simulink model "scd3busMicrogridDroopControlFidelityLevels"  (R2025b)
settings: Solver=ode15s  StartTime=0.0  StopTime=48  RelTol=1e-3
PreLoadFcn:
  | scd3busMicrogridDroopControlDataFidelityLevels;
  | 
  | %% Controller variants
  | % Create variant controls for converter controller. Controller has two
  | % different levels of fidelity: Averaged, AveragedPulse, Pulse
  | Averaged = Simulink.VariantExpression;
  | Averaged.Condition = 'fidelity==scd3busMicrogridDroopControl_variants_enum.Low';
  | Pulse = Simulink.VariantExpression;
  | Pulse.Condition = 'fidelity==scd3busMicrogridDroopControl_variants_enum.High';
  | 
  | %% Plant variants
  | % Create variant controls for converter plant. Plant has three different
  | % levels of fidelity.
  | AveragedNonSwitch = Simulink.VariantExpression;
  | AveragedNonSwitch.Condition = 'fidelity==scd3busMicrogridDroopControl_variants_enum.Low';
  | PulseSwitch = Simulink.VariantExpression;
  | PulseSwitch.Condition = 'fidelity==scd3busMicrogridDroopControl_variants_enum.High';
  | 
  | %% Set up variables ready for simulation
  | fidelity = scd3busMicrogridDroopControl_variants_enum.High;
  | Ts = 5e-6;
  | Ts_V = 1e-6;
  | Tsc = 1e-4;
  | Tsc_V = 5e-4;
values from neighbouring files (symbols this model uses):
  consensus = 1    [scd3busMicrogridDroopControlDataFidelityLevels.m]
  fgrid = 60    [scd3busMicrogridDroopControlDataFidelityLevels.m]    (also in scd3busMicrogridDroopControlDataFidelityLevels3Inv.m)
  Kdroop_fp = 0.02/2    (= 0.01)    [scd3busMicrogridDroopControlDataFidelityLevels.m]
  Kdroop_vq = 0.02/2    (= 0.01)    [scd3busMicrogridDroopControlDataFidelityLevels.m]
  Ki_vd = 850    [scd3busMicrogridDroopControlDataFidelityLevels.m]    (also in scd3busMicrogridDroopControlDataFidelityLevels3Inv.m)
  Ki_vq = 850    [scd3busMicrogridDroopControlDataFidelityLevels.m]    (also in scd3busMicrogridDroopControlDataFidelityLevels3Inv.m)
  Kp_vd = 0.36    [scd3busMicrogridDroopControlDataFidelityLevels.m]    (also in scd3busMicrogridDroopControlDataFidelityLevels3Inv.m)
  Kp_vq = 0.36    [scd3busMicrogridDroopControlDataFidelityLevels.m]    (also in scd3busMicrogridDroopControlDataFidelityLevels3Inv.m)
  Ts_DC = 0.001    [scd3busMicrogridDroopControlDataFidelityLevels.m]    (also in scd3busMicrogridDroopControlDataFidelityLevels3Inv.m = 0.0001)
  Vdc1 = 1000    [scd3busMicrogridDroopControlDataFidelityLevels.m]    (also in scd3busMicrogridDroopControlDataFidelityLevels3Inv.m)
  Vdc2 = 1000    [scd3busMicrogridDroopControlDataFidelityLevels.m]    (also in scd3busMicrogridDroopControlDataFidelityLevels3Inv.m)
  Vrms = 380    [scd3busMicrogridDroopControlDataFidelityLevels.m]    (also in scd3busMicrogridDroopControlDataFidelityLevels3Inv.m)
libraries: nesl_utility x60, ee_lib x57, fl_lib x32, eeTransforms x8, eeSinusoidalMeasurement x8, slpidlib x8, eePwmGeneratorTwoLevel x4, eePowerMeasurement x4, simulink x4, SignalEditorBlockLib x1
(part 2 of 5)

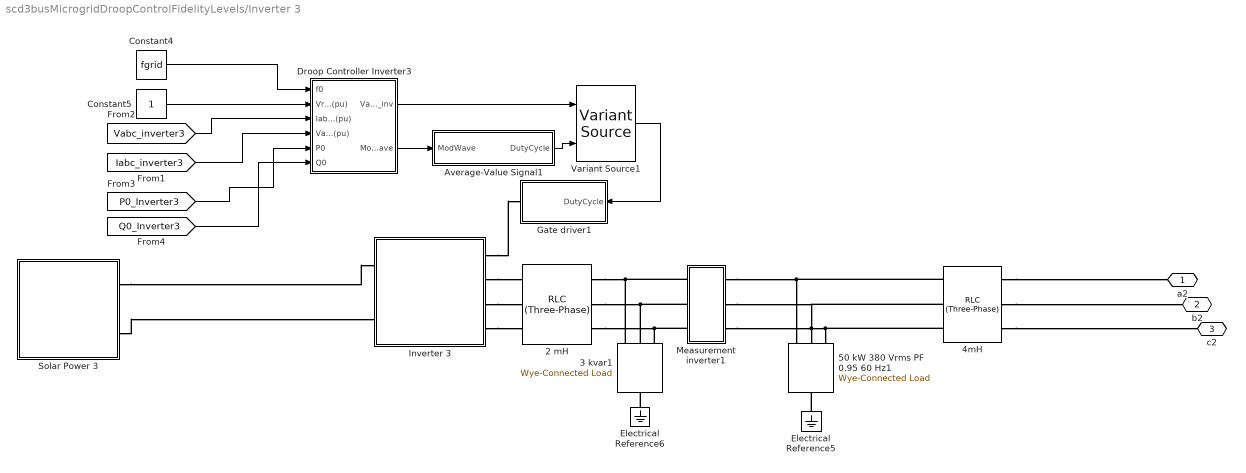
== system scd3busMicrogridDroopControlFidelityLevels/Inverter 3 ==
  2 mH : ee_lib/Passive/RLC Assemblies/RLC (Three-Phase)  port_option=ee.enum.threePhasePort.expanded  component_structure=ee.enum.rlc.structure.SeriesRL  R=0.02 Ohm  L=0.002 H  C=1 F  R_parasitic=1e-6 Ohm  G_parasitic=1e-6 1/Ohm  IL_specify=on  IL_priority=High  IL=[0, 0, 0] A  IL_nominal_specify=off  IL_nominal_value=1  IL_nominal_unit=A  VC_specify=on  VC_priority=High  VC=[0, 0, 0] V  VC_nominal_specify=off  VC_nominal_value=1  VC_nominal_unit=V
      settings: InternalSimscapePortConfiguration="{\"Bottom\":[],\"Left\":[{\"id\":\"a1\",\"label\":\"a1\",\"type\":\"foundation.electrical.electrical\"},{\"id\":\"b1\",\"label\":\"b1\",\"type\":\"foundation.electrical.electrical\"},{\"id\":\"c1\",\"label\":\"c1\",\"type\":\"foundation.electrical.electrical\"}],\"Right\":[{\"id\":\"a2\",\"label\":\"a2\",\"type\":\"foundation.electrical.electrical\"},{\"id\":\"b2\",\"label\":\"b2\",\"type\":\"foundation.electrical.electrical\"},{\"id\":\"c2\",\"label\":\"c2\",\"type\":\"foundation.electrical.electrical\"}],\"Top\":[]}"
  3 kvar1 : ee_lib/Passive/RLC Assemblies/Wye-Connected Load  port_option=ee.enum.threePhasePort.expanded  parameterization=ee.enum.rlc.parameterization.ratedpower  component_structure=ee.enum.rlc.structure.C  component_structure_PQ=ee.enum.rlc.structure.C  R=1 Ohm  L=0.001 H  C=1e-6 F  VRated=Vrms V  FRated=fgrid Hz  P=0 W  Qpos=0 A*V  Qneg=-3000 A*V  R_parasitic=1e-6 Ohm  G_parasitic=1e-6 1/Ohm  R_parasitic_PQ=1e-6 Ohm  G_parasitic_PQ=1e-6 1/Ohm  Vmag0=380 V  Vang0=0 deg  Freq0=60 Hz  IL_specify=on  IL_priority=High  IL=[ 0 0 0 ] A  IL_nominal_specify=off  IL_nominal_value=1  IL_nominal_unit=A  VC_specify=on  VC_priority=High  VC=[ 0 0 0 ] V  VC_nominal_specify=off  VC_nominal_value=1  VC_nominal_unit=V
      settings: InternalSimscapePortConfiguration="{\"Bottom\":[],\"Left\":[{\"id\":\"a\",\"label\":\"a\",\"type\":\"foundation.electrical.electrical\"},{\"id\":\"b\",\"label\":\"b\",\"type\":\"foundation.electrical.electrical\"},{\"id\":\"c\",\"label\":\"c\",\"type\":\"foundation.electrical.electrical\"}],\"Right\":[{\"id\":\"n\",\"label\":\"n\",\"type\":\"foundation.electrical.electrical\"}],\"Top\":[]}"
  "4mH " : ee_lib/Passive/RLC Assemblies/RLC (Three-Phase)  port_option=ee.enum.threePhasePort.expanded  component_structure=ee.enum.rlc.structure.SeriesRL  R=0.025 Ohm  L=0.004 H  C=1 F  R_parasitic=1e-6 Ohm  G_parasitic=1e-6 1/Ohm  IL_specify=on  IL_priority=High  IL=[0, 0, 0] A  IL_nominal_specify=off  IL_nominal_value=1  IL_nominal_unit=A  VC_specify=on  VC_priority=High  VC=[0, 0, 0] V  VC_nominal_specify=off  VC_nominal_value=1  VC_nominal_unit=V
      settings: InternalSimscapePortConfiguration="{\"Bottom\":[],\"Left\":[{\"id\":\"a1\",\"label\":\"a1\",\"type\":\"foundation.electrical.electrical\"},{\"id\":\"b1\",\"label\":\"b1\",\"type\":\"foundation.electrical.electrical\"},{\"id\":\"c1\",\"label\":\"c1\",\"type\":\"foundation.electrical.electrical\"}],\"Right\":[{\"id\":\"a2\",\"label\":\"a2\",\"type\":\"foundation.electrical.electrical\"},{\"id\":\"b2\",\"label\":\"b2\",\"type\":\"foundation.electrical.electrical\"},{\"id\":\"c2\",\"label\":\"c2\",\"type\":\"foundation.electrical.electrical\"}],\"Top\":[]}"
  50 kW 380 Vrms PF 0.95 60 Hz1 : ee_lib/Passive/RLC Assemblies/Wye-Connected Load  port_option=ee.enum.threePhasePort.expanded  parameterization=2  component_structure=1  component_structure_PQ=ee.enum.rlc.structure.ParallelRL  R=1 Ohm  L=0.001 H  C=1e-6 F  VRated=Vrms V  FRated=fgrid Hz  P=50000 W  Qpos=50000*sqrt(1-0.95^2)/0.95 V*A  Qneg=-3000 V*A  R_parasitic=1e-6 Ohm  G_parasitic=1e-6 1/Ohm  R_parasitic_PQ=1e-6 Ohm  G_parasitic_PQ=1e-6 1/Ohm  Vmag0=380 V  Vang0=0 deg  Freq0=60 Hz  IL_specify=on  IL_priority=High  IL=[ 0 0 0 ] A  IL_nominal_specify=off  IL_nominal_value=1  IL_nominal_unit=A  VC_specify=on  VC_priority=High  VC=[ 0 0 0 ] V  VC_nominal_specify=off  VC_nominal_value=1  VC_nominal_unit=V
      settings: InternalSimscapePortConfiguration="{\"Bottom\":[],\"Left\":[{\"id\":\"a\",\"label\":\"a\",\"type\":\"foundation.electrical.electrical\"},{\"id\":\"b\",\"label\":\"b\",\"type\":\"foundation.electrical.electrical\"},{\"id\":\"c\",\"label\":\"c\",\"type\":\"foundation.electrical.electrical\"}],\"Right\":[{\"id\":\"n\",\"label\":\"n\",\"type\":\"foundation.electrical.electrical\"}],\"Top\":[]}"
  Average-Value Signal1 : Subsystem
  Constant4 : Constant  Value=fgrid
  Constant5 : Constant
  Droop Controller Inverter3 : Subsystem
  Electrical Reference5 : fl_lib/Electrical/Electrical Elements/Electrical Reference
  Electrical Reference6 : fl_lib/Electrical/Electrical Elements/Electrical Reference
  Gate driver1 : Subsystem
  Inverter 3 : Subsystem  Variant=on  VariantControl=Choice
  Measurement inverter1 : Subsystem
  Solar Power 3 : Subsystem
  Variant Source1 : VariantSource  ShowConditionOnBlock=on  VariantControls={Pulse, Averaged}
  a2 : PMIOPort  Side=Right
  b2 : PMIOPort  Port=2  Side=Right
  c2 : PMIOPort  Port=3  Side=Right
  wires:
  Variant Source1/1 -> Gate driver1/1(DutyCycle)
  Droop Controller Inverter3/2(ModWave) -> Average-Value Signal1/1(ModWave)
  [P0_Inverter3] -> Droop Controller Inverter3/5(P0)
  [Vabc_inverter3] -> Droop Controller Inverter3/3(Iabc (pu))
  Constant4/1 -> Droop Controller Inverter3/1(f0)
  Constant5/1 -> Droop Controller Inverter3/2(Vref (pu))
  [Iabc_inverter3] -> Droop Controller Inverter3/4(Vabc (pu))
  Droop Controller Inverter3/1(Vabc_inv) -> Variant Source1/1
  [Q0_Inverter3] -> Droop Controller Inverter3/6(Q0)
  Average-Value Signal1/1(DutyCycle) -> Variant Source1/2
  connections:
  50 kW 380 Vrms PF 0.95 60 Hz1/LConn2 -- Measurement inverter1/RConn2 -- "4mH "/LConn2
  50 kW 380 Vrms PF 0.95 60 Hz1/LConn3 -- Measurement inverter1/RConn3 -- "4mH "/LConn3
  "4mH "/RConn1 -- a2/RConn1
  Inverter 3/LConn3 -- 2 mH/LConn2
  "4mH "/LConn1 -- Measurement inverter1/RConn1 -- 50 kW 380 Vrms PF 0.95 60 Hz1/LConn1
  Solar Power 3/RConn2 -- Inverter 3/RConn2
  "4mH "/RConn3 -- c2/RConn1
  Electrical Reference6/LConn1 -- 3 kvar1/RConn1
  Inverter 3/LConn4 -- 2 mH/LConn3
  "4mH "/RConn2 -- b2/RConn1
  Electrical Reference5/LConn1 -- 50 kW 380 Vrms PF 0.95 60 Hz1/RConn1
  2 mH/RConn2 -- Measurement inverter1/LConn2 -- 3 kvar1/LConn2
  2 mH/RConn3 -- Measurement inverter1/LConn3 -- 3 kvar1/LConn3
  Solar Power 3/RConn1 -- Inverter 3/RConn1
  2 mH/RConn1 -- Measurement inverter1/LConn1 -- 3 kvar1/LConn1
  Inverter 3/LConn2 -- 2 mH/LConn1
  Inverter 3/LConn1 -- Gate driver1/RConn1

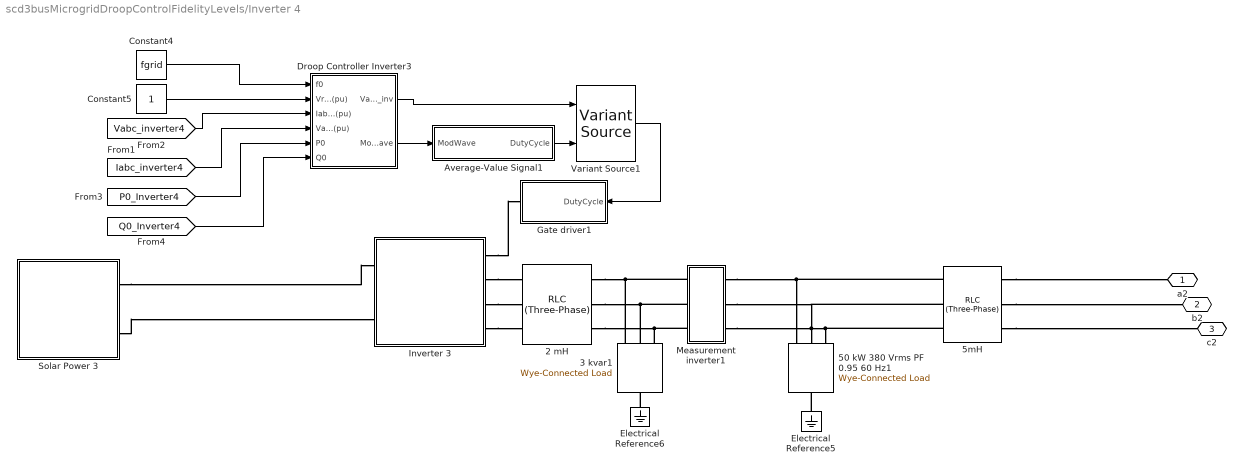
== system scd3busMicrogridDroopControlFidelityLevels/Inverter 4 ==
  2 mH : ee_lib/Passive/RLC Assemblies/RLC (Three-Phase)  port_option=ee.enum.threePhasePort.expanded  component_structure=ee.enum.rlc.structure.SeriesRL  R=0.02 Ohm  L=0.002 H  C=1 F  R_parasitic=1e-6 Ohm  G_parasitic=1e-6 1/Ohm  IL_specify=on  IL_priority=High  IL=[0, 0, 0] A  IL_nominal_specify=off  IL_nominal_value=1  IL_nominal_unit=A  VC_specify=on  VC_priority=High  VC=[0, 0, 0] V  VC_nominal_specify=off  VC_nominal_value=1  VC_nominal_unit=V
      settings: InternalSimscapePortConfiguration="{\"Bottom\":[],\"Left\":[{\"id\":\"a1\",\"label\":\"a1\",\"type\":\"foundation.electrical.electrical\"},{\"id\":\"b1\",\"label\":\"b1\",\"type\":\"foundation.electrical.electrical\"},{\"id\":\"c1\",\"label\":\"c1\",\"type\":\"foundation.electrical.electrical\"}],\"Right\":[{\"id\":\"a2\",\"label\":\"a2\",\"type\":\"foundation.electrical.electrical\"},{\"id\":\"b2\",\"label\":\"b2\",\"type\":\"foundation.electrical.electrical\"},{\"id\":\"c2\",\"label\":\"c2\",\"type\":\"foundation.electrical.electrical\"}],\"Top\":[]}"
  3 kvar1 : ee_lib/Passive/RLC Assemblies/Wye-Connected Load  port_option=ee.enum.threePhasePort.expanded  parameterization=ee.enum.rlc.parameterization.ratedpower  component_structure=ee.enum.rlc.structure.C  component_structure_PQ=ee.enum.rlc.structure.C  R=1 Ohm  L=0.001 H  C=1e-6 F  VRated=Vrms V  FRated=fgrid Hz  P=0 W  Qpos=0 A*V  Qneg=-3000 A*V  R_parasitic=1e-6 Ohm  G_parasitic=1e-6 1/Ohm  R_parasitic_PQ=1e-6 Ohm  G_parasitic_PQ=1e-6 1/Ohm  Vmag0=380 V  Vang0=0 deg  Freq0=60 Hz  IL_specify=on  IL_priority=High  IL=[ 0 0 0 ] A  IL_nominal_specify=off  IL_nominal_value=1  IL_nominal_unit=A  VC_specify=on  VC_priority=High  VC=[ 0 0 0 ] V  VC_nominal_specify=off  VC_nominal_value=1  VC_nominal_unit=V
      settings: InternalSimscapePortConfiguration="{\"Bottom\":[],\"Left\":[{\"id\":\"a\",\"label\":\"a\",\"type\":\"foundation.electrical.electrical\"},{\"id\":\"b\",\"label\":\"b\",\"type\":\"foundation.electrical.electrical\"},{\"id\":\"c\",\"label\":\"c\",\"type\":\"foundation.electrical.electrical\"}],\"Right\":[{\"id\":\"n\",\"label\":\"n\",\"type\":\"foundation.electrical.electrical\"}],\"Top\":[]}"
  50 kW 380 Vrms PF 0.95 60 Hz1 : ee_lib/Passive/RLC Assemblies/Wye-Connected Load  port_option=ee.enum.threePhasePort.expanded  parameterization=2  component_structure=1  component_structure_PQ=ee.enum.rlc.structure.ParallelRL  R=1 Ohm  L=0.001 H  C=1e-6 F  VRated=Vrms V  FRated=fgrid Hz  P=50000 W  Qpos=50000*sqrt(1-0.95^2)/0.95 V*A  Qneg=-3000 V*A  R_parasitic=1e-6 Ohm  G_parasitic=1e-6 1/Ohm  R_parasitic_PQ=1e-6 Ohm  G_parasitic_PQ=1e-6 1/Ohm  Vmag0=380 V  Vang0=0 deg  Freq0=60 Hz  IL_specify=on  IL_priority=High  IL=[ 0 0 0 ] A  IL_nominal_specify=off  IL_nominal_value=1  IL_nominal_unit=A  VC_specify=on  VC_priority=High  VC=[ 0 0 0 ] V  VC_nominal_specify=off  VC_nominal_value=1  VC_nominal_unit=V
      settings: InternalSimscapePortConfiguration="{\"Bottom\":[],\"Left\":[{\"id\":\"a\",\"label\":\"a\",\"type\":\"foundation.electrical.electrical\"},{\"id\":\"b\",\"label\":\"b\",\"type\":\"foundation.electrical.electrical\"},{\"id\":\"c\",\"label\":\"c\",\"type\":\"foundation.electrical.electrical\"}],\"Right\":[{\"id\":\"n\",\"label\":\"n\",\"type\":\"foundation.electrical.electrical\"}],\"Top\":[]}"
  "5mH " : ee_lib/Passive/RLC Assemblies/RLC (Three-Phase)  port_option=ee.enum.threePhasePort.expanded  component_structure=ee.enum.rlc.structure.SeriesRL  R=0.005 Ohm  L=0.002 H  C=1 F  R_parasitic=1e-6 Ohm  G_parasitic=1e-6 1/Ohm  IL_specify=on  IL_priority=High  IL=[0, 0, 0] A  IL_nominal_specify=off  IL_nominal_value=1  IL_nominal_unit=A  VC_specify=on  VC_priority=High  VC=[0, 0, 0] V  VC_nominal_specify=off  VC_nominal_value=1  VC_nominal_unit=V
      settings: InternalSimscapePortConfiguration="{\"Bottom\":[],\"Left\":[{\"id\":\"a1\",\"label\":\"a1\",\"type\":\"foundation.electrical.electrical\"},{\"id\":\"b1\",\"label\":\"b1\",\"type\":\"foundation.electrical.electrical\"},{\"id\":\"c1\",\"label\":\"c1\",\"type\":\"foundation.electrical.electrical\"}],\"Right\":[{\"id\":\"a2\",\"label\":\"a2\",\"type\":\"foundation.electrical.electrical\"},{\"id\":\"b2\",\"label\":\"b2\",\"type\":\"foundation.electrical.electrical\"},{\"id\":\"c2\",\"label\":\"c2\",\"type\":\"foundation.electrical.electrical\"}],\"Top\":[]}"
  Average-Value Signal1 : Subsystem
  Constant4 : Constant  Value=fgrid
  Constant5 : Constant
  Droop Controller Inverter3 : Subsystem
  Electrical Reference5 : fl_lib/Electrical/Electrical Elements/Electrical Reference
  Electrical Reference6 : fl_lib/Electrical/Electrical Elements/Electrical Reference
  Gate driver1 : Subsystem
  Inverter 3 : Subsystem  Variant=on  VariantControl=Choice
  Measurement inverter1 : Subsystem
  Solar Power 3 : Subsystem
  Variant Source1 : VariantSource  ShowConditionOnBlock=on  VariantControls={Pulse, Averaged}
  a2 : PMIOPort  Side=Right
  b2 : PMIOPort  Port=2  Side=Right
  c2 : PMIOPort  Port=3  Side=Right
  wires:
  Variant Source1/1 -> Gate driver1/1(DutyCycle)
  Droop Controller Inverter3/2(ModWave) -> Average-Value Signal1/1(ModWave)
  [P0_Inverter4] -> Droop Controller Inverter3/5(P0)
  [Vabc_inverter4] -> Droop Controller Inverter3/3(Iabc (pu))
  Constant4/1 -> Droop Controller Inverter3/1(f0)
  Constant5/1 -> Droop Controller Inverter3/2(Vref (pu))
  [Iabc_inverter4] -> Droop Controller Inverter3/4(Vabc (pu))
  Droop Controller Inverter3/1(Vabc_inv) -> Variant Source1/1
  [Q0_Inverter4] -> Droop Controller Inverter3/6(Q0)
  Average-Value Signal1/1(DutyCycle) -> Variant Source1/2
  connections:
  50 kW 380 Vrms PF 0.95 60 Hz1/LConn2 -- Measurement inverter1/RConn2 -- "5mH "/LConn2
  50 kW 380 Vrms PF 0.95 60 Hz1/LConn3 -- Measurement inverter1/RConn3 -- "5mH "/LConn3
  "5mH "/RConn1 -- a2/RConn1
  Inverter 3/LConn3 -- 2 mH/LConn2
  "5mH "/LConn1 -- Measurement inverter1/RConn1 -- 50 kW 380 Vrms PF 0.95 60 Hz1/LConn1
  Solar Power 3/RConn2 -- Inverter 3/RConn2
  "5mH "/RConn3 -- c2/RConn1
  Electrical Reference6/LConn1 -- 3 kvar1/RConn1
  Inverter 3/LConn4 -- 2 mH/LConn3
  "5mH "/RConn2 -- b2/RConn1
  Electrical Reference5/LConn1 -- 50 kW 380 Vrms PF 0.95 60 Hz1/RConn1
  2 mH/RConn2 -- Measurement inverter1/LConn2 -- 3 kvar1/LConn2
  2 mH/RConn3 -- Measurement inverter1/LConn3 -- 3 kvar1/LConn3
  Solar Power 3/RConn1 -- Inverter 3/RConn1
  2 mH/RConn1 -- Measurement inverter1/LConn1 -- 3 kvar1/LConn1
  Inverter 3/LConn2 -- 2 mH/LConn1
  Inverter 3/LConn1 -- Gate driver1/RConn1

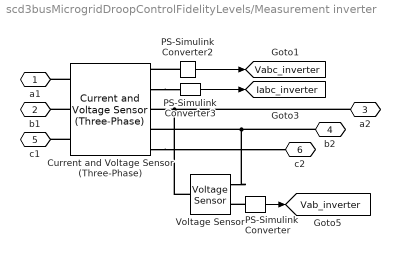
== system scd3busMicrogridDroopControlFidelityLevels/Measurement inverter ==
  Current and Voltage Sensor (Three-Phase) : ee_lib/Sensors & Transducers/Current and Voltage Sensor (Three-Phase)  vMeasurementType=2  outputUnit=1  SRated=150000 V*A  VRated=Vrms V  I_specify=off  I_priority=None  I=[ 0 0 0 ] A  I_nominal_specify=off  I_nominal_value=1  I_nominal_unit=A  V_specify=off  V_priority=None  V=[ 0 0 0 ] V  V_nominal_specify=off  V_nominal_value=1  V_nominal_unit=V
      settings: InternalSimscapePortConfiguration="{\"Bottom\":[],\"Left\":[{\"id\":\"a1\",\"label\":\"a1\",\"type\":\"foundation.electrical.electrical\"},{\"id\":\"b1\",\"label\":\"b1\",\"type\":\"foundation.electrical.electrical\"},{\"id\":\"c1\",\"label\":\"c1\",\"type\":\"foundation.electrical.electrical\"}],\"Right\":[{\"id\":\"V_output\",\"label\":\"V\",\"type\":\"output\"},{\"id\":\"I_output\",\"label\":\"I\",\"type\":\"output\"},{\"id\":\"a2\",\"label\":\"a2\",\"type\":\"foundation.electrical.electrical\"},{\"id\":\"b2\",\"label\":\"b2\",\"type\":\"foundation.electrical.electrical\"},{\"id\":\"c2\",\"label\":\"c2\",\"type\":\"foundation.electrical.electrical\"}],\"Top\":[]}"
  PS-Simulink Converter : nesl_utility/PS-Simulink Converter  PhysicalDomain=network_engine_domain  SubClassName=ps_output  LeftPortType=input  RightPortType=output  PseudoPeriodic=off  Frequencies=[]  VectorFormat=1-D array  Unit=V  AffineConversion=off
  PS-Simulink Converter2 : nesl_utility/PS-Simulink Converter  PhysicalDomain=network_engine_domain  SubClassName=ps_output  LeftPortType=input  RightPortType=output  PseudoPeriodic=off  Frequencies=[]  VectorFormat=1-D array  Unit=1  AffineConversion=off
  PS-Simulink Converter3 : nesl_utility/PS-Simulink Converter  PhysicalDomain=network_engine_domain  SubClassName=ps_output  LeftPortType=input  RightPortType=output  PseudoPeriodic=off  Frequencies=[]  VectorFormat=1-D array  Unit=1  AffineConversion=off
  Voltage Sensor : fl_lib/Electrical/Electrical Sensors/Voltage Sensor
  a1 : PMIOPort  Side=Left
  b1 : PMIOPort  Port=2  Side=Left
  a2 : PMIOPort  Port=3  Side=Right
  b2 : PMIOPort  Port=4  Side=Right
  c1 : PMIOPort  Port=5  Side=Left
  c2 : PMIOPort  Port=6  Side=Right
  tag scope: Iabc_inverter=global, Vab_inverter=global, Vabc_inverter=global
  wires:
  PS-Simulink Converter2/1 -> [Vabc_inverter]
  PS-Simulink Converter3/1 -> [Iabc_inverter]
  PS-Simulink Converter/1 -> [Vab_inverter]
  connections:
  b2/RConn1 -- Voltage Sensor/RConn2 -- Current and Voltage Sensor (Three-Phase)/RConn4
  a2/RConn1 -- Voltage Sensor/LConn1 -- Current and Voltage Sensor (Three-Phase)/RConn3
  Current and Voltage Sensor (Three-Phase)/RConn5 -- c2/RConn1
  Current and Voltage Sensor (Three-Phase)/LConn2 -- b1/RConn1
  Current and Voltage Sensor (Three-Phase)/LConn3 -- c1/RConn1
  Current and Voltage Sensor (Three-Phase)/LConn1 -- a1/RConn1
  PS-Simulink Converter2/LConn1 -- Current and Voltage Sensor (Three-Phase)/RConn1
  Current and Voltage Sensor (Three-Phase)/RConn2 -- PS-Simulink Converter3/LConn1
  PS-Simulink Converter/LConn1 -- Voltage Sensor/RConn1

== system scd3busMicrogridDroopControlFidelityLevels/Operation Commands ==
  Microgrid Operation Scheduler : SignalEditorBlockLib/Signal Editor  FileName=scd3busMicrogridDroopControlSetPoints.mat  ActiveScenario=Scenario  ActiveSignal=P_inverter2  IsBus=off  OutputBusObjectStr=Bus: BusObject  SampleTime=0  Interpolate=off  ZeroCross=off  OutputAfterFinalValue=Setting to zero  Unit=inherit  PreserveSignalName=on  ApplySigPropsToAllScenarios=on  ApplySigPropsToAllSignals=off  SignalPropertySource=Dialog parameters
  tag scope: P0_Inverter1=global, P0_Inverter2=global, P0_Inverter3=global, P0_Inverter4=global, Q0_Inverter1=global, Q0_Inverter2=global, Q0_Inverter3=global, Q0_Inverter4=global
  wires:
  Microgrid Operation Scheduler/4 -> [Q0_Inverter2]
  Microgrid Operation Scheduler/1 -> [P0_Inverter1]
  Microgrid Operation Scheduler/3 -> [P0_Inverter2]
  Microgrid Operation Scheduler/2 -> [Q0_Inverter1]
  Microgrid Operation Scheduler/5 -> [P0_Inverter3]
  Microgrid Operation Scheduler/6 -> [Q0_Inverter3]
  Microgrid Operation Scheduler/7 -> [P0_Inverter4]
  Microgrid Operation Scheduler/8 -> [Q0_Inverter4]

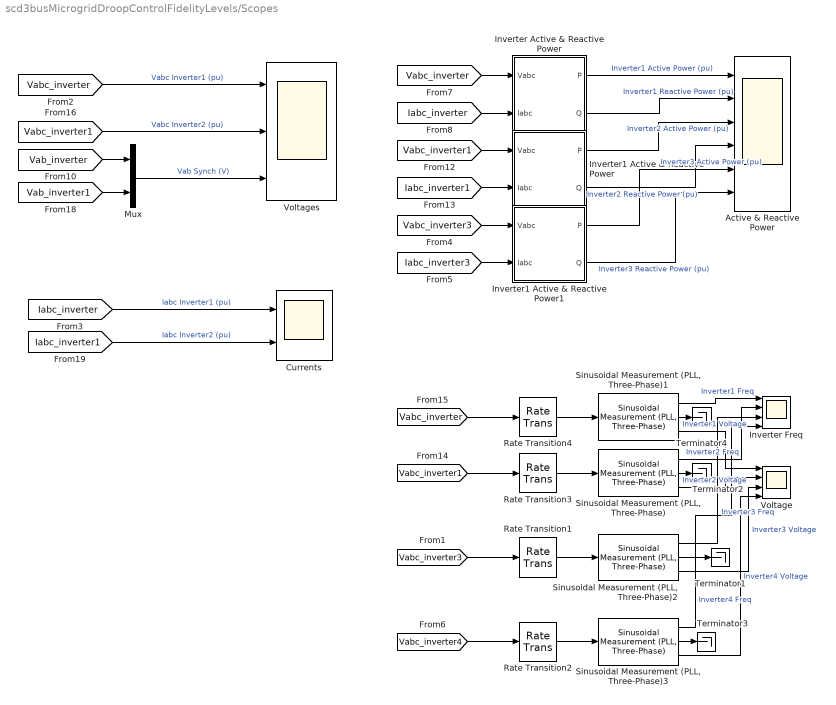
== system scd3busMicrogridDroopControlFidelityLevels/Scopes ==
  Active & Reactive Power : Scope  NumInputPorts=6
      settings: ActiveDisplayString=4  ActiveDisplayYMinimum=-2.1984157786569289  ActiveDisplayYMaximum=3.1037614802677909  DataLoggingDecimation=10
  Currents : Scope  NumInputPorts=2
      settings: ActiveDisplayYMinimum=-1.1087  ActiveDisplayYMaximum=1.10389  DataLoggingVariableName=ScopeData2
  "Inverter Active & Reactive Power " : Subsystem
  Inverter Freq : Scope  NumInputPorts=4
      settings: ActiveDisplayYMinimum=56.727408569108626  ActiveDisplayYMaximum=67.198343596660337  DataLoggingVariableName=ScopeData2
  Inverter1 Active & Reactive Power : Subsystem
  Inverter1 Active & Reactive Power1 : Subsystem
  Mux : Mux  Inputs=2
  Rate Transition{1..4} (4 alike) : RateTransition  OutPortSampleTime=Tsc
  Sinusoidal Measurement (PLL, Three-Phase){,1..3} (4 alike) : eeSinusoidalMeasurement/Sinusoidal Measurement (PLL, Three-Phase)  Kp_LF=150  Ki_LF=150  F0=fgrid  Theta0=0  Ts=Tsc
  Terminator{1..4} (4 alike) : Terminator
  Voltage : Scope  NumInputPorts=4
      settings: ActiveDisplayYMinimum=-0.15968079072818678  ActiveDisplayYMaximum=1.4634228980026596
  Voltages : Scope  NumInputPorts=3
      settings: ActiveDisplayYMinimum=-1.3151  ActiveDisplayYMaximum=1.31718  DataLoggingVariableName=ScopeData6
  wires:
  [Iabc_inverter] -> Currents/1  "Iabc Inverter1 (pu)"
  [Vabc_inverter] -> Voltages/1  "Vabc Inverter1 (pu)"
  [Vabc_inverter] -> "Inverter Active & Reactive Power "/1(Vabc)
  [Iabc_inverter] -> "Inverter Active & Reactive Power "/2(Iabc)
  "Inverter Active & Reactive Power "/1(P) -> Active & Reactive Power/1  "Inverter1 Active Power (pu)"
  Mux/1 -> Voltages/3  "Vab Synch (V)"
  [Vab_inverter] -> Mux/1
  "Inverter Active & Reactive Power "/2(Q) -> Active & Reactive Power/2  "Inverter1 Reactive Power (pu)"
  Inverter1 Active & Reactive Power/2(Q) -> Active & Reactive Power/4  "Inverter2 Reactive Power (pu)"
  Inverter1 Active & Reactive Power/1(P) -> Active & Reactive Power/3  "Inverter2 Active Power (pu)"
  [Iabc_inverter1] -> Inverter1 Active & Reactive Power/2(Iabc)
  [Vabc_inverter1] -> Inverter1 Active & Reactive Power/1(Vabc)
  Rate Transition3/1 -> "Sinusoidal Measurement (PLL, Three-Phase)"/1
  "Sinusoidal Measurement (PLL, Three-Phase)"/1 -> Inverter Freq/2  "Inverter2 Freq"
  Rate Transition4/1 -> "Sinusoidal Measurement (PLL, Three-Phase)1"/1
  "Sinusoidal Measurement (PLL, Three-Phase)1"/2 -> Terminator4/1
  "Sinusoidal Measurement (PLL, Three-Phase)1"/1 -> Inverter Freq/1  "Inverter1 Freq"
  [Vabc_inverter] -> Rate Transition4/1
  "Sinusoidal Measurement (PLL, Three-Phase)"/2 -> Terminator2/1
  [Vabc_inverter1] -> Rate Transition3/1
  "Sinusoidal Measurement (PLL, Three-Phase)"/3 -> Voltage/2  "Inverter2 Voltage"
  "Sinusoidal Measurement (PLL, Three-Phase)1"/3 -> Voltage/1  "Inverter1 Voltage"
  [Vab_inverter1] -> Mux/2
  [Iabc_inverter1] -> Currents/2  "Iabc Inverter2 (pu)"
  [Vabc_inverter1] -> Voltages/2  "Vabc Inverter2 (pu)"
  Rate Transition1/1 -> "Sinusoidal Measurement (PLL, Three-Phase)2"/1
  [Vabc_inverter3] -> Rate Transition1/1
  "Sinusoidal Measurement (PLL, Three-Phase)2"/1 -> Inverter Freq/3  "Inverter3 Freq"
  "Sinusoidal Measurement (PLL, Three-Phase)2"/2 -> Terminator1/1
  "Sinusoidal Measurement (PLL, Three-Phase)2"/3 -> Voltage/3  "Inverter3 Voltage"
  [Vabc_inverter3] -> Inverter1 Active & Reactive Power1/1(Vabc)
  [Iabc_inverter3] -> Inverter1 Active & Reactive Power1/2(Iabc)
  Inverter1 Active & Reactive Power1/1(P) -> Active & Reactive Power/5  "Inverter3 Active Power (pu)"
  Inverter1 Active & Reactive Power1/2(Q) -> Active & Reactive Power/6  "Inverter3 Reactive Power (pu)"
  Rate Transition2/1 -> "Sinusoidal Measurement (PLL, Three-Phase)3"/1
  [Vabc_inverter4] -> Rate Transition2/1
  "Sinusoidal Measurement (PLL, Three-Phase)3"/1 -> Inverter Freq/4  "Inverter4 Freq"
  "Sinusoidal Measurement (PLL, Three-Phase)3"/3 -> Voltage/4  "Inverter4 Voltage"
  "Sinusoidal Measurement (PLL, Three-Phase)3"/2 -> Terminator3/1

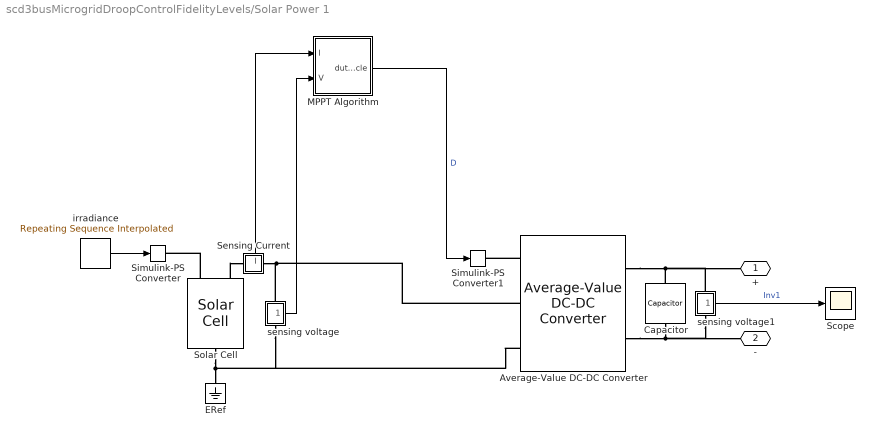
== system scd3busMicrogridDroopControlFidelityLevels/Solar Power 1 ==
  Average-Value DC-DC Converter : ee_lib/Semiconductors & Converters/Converters/Average-Value DC-DC Converter  implementation_option=ee.enum.converters.implementation.behavioral  converter_type=ee.enum.converters.dcdctype.buckboost  control_option=ee.enum.converters.controlinput.dutycycle  efficiency_option=ee.enum.converters.efficiency.constant  efficiency_fixed=100  i_vec=[0, 2, 5] A  efficiency_vec=[90, 95, 98]  Lf=1e-6 H  Rl=0 Ohm  Cf=1e-7 F  Rc=1e-6 Ohm  iL_specify=off  iL_priority=High  iL=0 A  iL_nominal_specify=off  iL_nominal_value=1  iL_nominal_unit=A  vc_specify=off  vc_priority=High  vc=0 V  vc_nominal_specify=off  vc_nominal_value=1  vc_nominal_unit=V
      settings: InternalSimscapePortConfiguration="{\"Bottom\":[],\"Left\":[{\"id\":\"DutyCycle\",\"label\":\"DutyCycle\",\"type\":\"input\"},{\"id\":\"p1\",\"label\":\"1+\",\"type\":\"foundation.electrical.electrical\"},{\"id\":\"n1\",\"label\":\"1-\",\"type\":\"foundation.electrical.electrical\"}],\"Right\":[{\"id\":\"p2\",\"label\":\"2+\",\"type\":\"foundation.electrical.electrical\"},{\"id\":\"n2\",\"label\":\"2-\",\"type\":\"foundation.electrical.electrical\"}],\"Top\":[]}"
  Capacitor : ee_lib/Passive/Capacitor  cap_option=ee.enum.passive.capacitor.capOption.const  c=2200e-6 F  Cvec=[1e-05, 1e-06] F  Vvec=[0, 10] V  CV_table_symmetry=ee.enum.passive.capacitor.tableSymmetry.yes  f_vec=[1, 10] kHz  DFext_vec=[.8, 1.2]  enable_C_tol=ee.enum.toleranceApplication.none  averaging_period=0 s  C_tol=5  tol_distribution=ee.enum.toleranceDistribution.uniform  nSigma=4  r=0 Ohm  g=0 1/Ohm  enable_operating_limits=ee.enum.enable.no  operating_limit_action=ee.enum.passive.reportOpLim.warn  max_working_voltage_range=[-25, 25] V  power_rating=1 W  maxTemperature=85 degC  thermalEnable=false  thermalMass=1 J/K  i_specify=off  i_priority=None  i=0 A  i_nominal_specify=off  i_nominal_value=1  i_nominal_unit=A  v_specify=off  v_priority=None  v=0 V  v_nominal_specify=off  v_nominal_value=1  v_nominal_unit=V  vc_specify=on  vc_priority=High  vc=1000 V  vc_nominal_specify=off  vc_nominal_value=1  vc_nominal_unit=V  T_specify=off  T_priority=None  T=298.15 K  T_nominal_specify=off  T_nominal_value=1  T_nominal_unit=K
  ERef : fl_lib/Electrical/Electrical Elements/Electrical Reference
  MPPT Algorithm : Subsystem
  Scope : Scope
      settings: ActiveDisplayYMinimum=404.36190016851077  ActiveDisplayYMaximum=1106.9912522955344
  Sensing Current : Subsystem
      settings: PortSchema="{\"entries\":[{\"content\":{\"sides\":[{\"content\":{\"connectorIds\":[\"LConn1\"]},\"type\":\"ConnectorPlacement.EquallySpacedRectSide\",\"uuid\":\"08eaf192-3836-4d70-9f6a-c3aee0977ea6\"},{\"content\":{\"connectorIds\":[\"RConn1\"],\"side\":\"RIGHT\"},\"type\":\"ConnectorPlacement.EquallySpacedRectSide\",\"uuid\":\"69615d36-c1bf-4d31-b3e4-77c73286e7c7\"},{\"content\":{\"connectorIds\":[\"Out1\"],\"side\":\"TOP\"},\"type\":\"ConnectorPlacement.EquallySpacedRectSide\",\"uuid\":\"21e31d90-f675-47e5-98f5-1bf7e6a5fdbe\"}]},\"type\":\"ConnectorPlacement.EquallySpacedConnector\",\"uuid\":\"068abd2e-abc9-41d7-b40e-d83d3e3b9346\"}],\"packageUris\":[\"http://schema.mathworks.com/mf0/Connector/R2020b\"],\"version\":\"1.0\"}"
      mask Display: disp('i')
  Simulink-PS Converter : nesl_utility/Simulink-PS Converter  PhysicalDomain=network_engine_domain  SubClassName=ps_input  LeftPortType=input  RightPortType=output  PseudoPeriodic=off  Frequencies=[]  NoiseDistribution=none  NoiseParameters=[]  Unit=1  AffineConversion=off  FilteringAndDerivatives=provide  SimscapeFilterOrder=1  InputFilterTimeConstant=0.001  UdotUserProvided=0
  Simulink-PS Converter1 : nesl_utility/Simulink-PS Converter  PhysicalDomain=network_engine_domain  SubClassName=ps_input  LeftPortType=input  RightPortType=output  PseudoPeriodic=off  Frequencies=[]  NoiseDistribution=none  NoiseParameters=[]  Unit=1  AffineConversion=off  FilteringAndDerivatives=provide  SimscapeFilterOrder=1  InputFilterTimeConstant=0.001  UdotUserProvided=0
  Solar Cell : ee_lib/Sources/Solar Cell  PartSpecification="{\"CollectionId\":\"SimscapeElectrical\",\"CollectionVersion\":\"1.0.0\",\"DatasetId\":\"Amerisolar|AS_6M_360W_PERC|simscape.electrical.solarCell\",\"DisplayName\":\"Amerisolar:AS_6M_360W_PERC\"}"  prm=3  Isc=9.64 % Datasheet derived A  Voc=0.65833 % Datasheet derived V  Is=3.26005689221038e-07 % Datasheet derived A  Is2=2.08812935747622e-09 % Datasheet derived A  Iph=9.64000663446818 % Datasheet derived A  Ir0=1000 % Datasheet derived W/m^2  ec=1.48955183509565 % Datasheet derived  N2=2.03537290915688 % Datasheet derived  Rs=0.000587128359683705 % Datasheet derived Ohm  Rp=771.966793824014 % Datasheet derived Ohm  N_series=10 * 72 % Datasheet derived  N_parallel=25 % Datasheet derived  TIPH1=0.000519981408860291 % Datasheet derived 1/K  EG=1.12 % Datasheet derived eV  TXIS1=4.17598231137541 % Datasheet derived  TXIS2=18.4602091098286 % Datasheet derived  TRS1=0.101104089054628 % Datasheet derived  TRP1=0 % Parameter not set  Tmeas=25 % Datasheet derived degC  TFIXED=25 % Datasheet derived degC  thermal_mass=100 % Parameter not set J/K  initial_temperature=25 degC
      settings: AttributesFormatString=Amerisolar:AS_6M_360W_PERC
  "irradiance " : simulink/Sources/Repeating Sequence Interpolated  OutValues=[5 5 5 5 5 5 5 5 5 5 5 5 5 5 5 5 5 5 5 5 5 5 5 5]*200  TimeValues=[0 1 2 3 4 5 6 7 8 9 10 11 12 13 14 15 16 17 18 19 20 21 22 23]  LookUpMeth=Interpolation-Use End Values  tsamp=0.001  OutMin=[]  OutMax=[]  OutDataTypeStr=double  OutputDataTypeScalingMode=double  OutDataType=fixdt(0,8)  OutScaling=2^-10
  sensing voltage : Subsystem
      settings: PortSchema="{\"entries\":[{\"content\":{\"sides\":[{\"content\":{\"connectorIds\":[\"LConn1\"]},\"type\":\"ConnectorPlacement.EquallySpacedRectSide\",\"uuid\":\"08eaf192-3836-4d70-9f6a-c3aee0977ea6\"},{\"content\":{\"connectorIds\":[\"RConn1\"],\"side\":\"RIGHT\"},\"type\":\"ConnectorPlacement.EquallySpacedRectSide\",\"uuid\":\"69615d36-c1bf-4d31-b3e4-77c73286e7c7\"},{\"content\":{\"connectorIds\":[],\"side\":\"TOP\"},\"type\":\"ConnectorPlacement.EquallySpacedRectSide\",\"uuid\":\"21e31d90-f675-47e5-98f5-1bf7e6a5fdbe\"},{\"content\":{\"connectorIds\":[\"Out1\"],\"side\":\"BOTTOM\"},\"type\":\"ConnectorPlacement.EquallySpacedRectSide\",\"uuid\":\"23a77980-6beb-4147-b48e-adf9e1983263\"}]},\"type\":\"ConnectorPlacement.EquallySpacedConnector\",\"uuid\":\"068abd2e-abc9-41d7-b40e-d83d3e3b9346\"}],\"packageUris\":[\"http://schema.mathworks.com/mf0/Connector/R2020b\"],\"version\":\"1.0\"}"
      mask Display: disp('v')
  sensing voltage1 : Subsystem
      settings: PortSchema="{\"entries\":[{\"content\":{\"sides\":[{\"content\":{\"connectorIds\":[\"LConn1\"]},\"type\":\"ConnectorPlacement.EquallySpacedRectSide\",\"uuid\":\"08eaf192-3836-4d70-9f6a-c3aee0977ea6\"},{\"content\":{\"connectorIds\":[\"RConn1\"],\"side\":\"RIGHT\"},\"type\":\"ConnectorPlacement.EquallySpacedRectSide\",\"uuid\":\"69615d36-c1bf-4d31-b3e4-77c73286e7c7\"},{\"content\":{\"connectorIds\":[],\"side\":\"TOP\"},\"type\":\"ConnectorPlacement.EquallySpacedRectSide\",\"uuid\":\"21e31d90-f675-47e5-98f5-1bf7e6a5fdbe\"},{\"content\":{\"connectorIds\":[\"Out1\"],\"side\":\"BOTTOM\"},\"type\":\"ConnectorPlacement.EquallySpacedRectSide\",\"uuid\":\"23a77980-6beb-4147-b48e-adf9e1983263\"}]},\"type\":\"ConnectorPlacement.EquallySpacedConnector\",\"uuid\":\"068abd2e-abc9-41d7-b40e-d83d3e3b9346\"}],\"packageUris\":[\"http://schema.mathworks.com/mf0/Connector/R2020b\"],\"version\":\"1.0\"}"
      mask Display: disp('v')
  + : PMIOPort  Side=Right
  - : PMIOPort  Port=2  Side=Right
  wires:
  sensing voltage/1(V) -> MPPT Algorithm/2(V)
  Sensing Current/1(I) -> MPPT Algorithm/1(I)
  MPPT Algorithm/1(duty_cycle) -> Simulink-PS Converter1/1  "D"
  "irradiance "/1 -> Simulink-PS Converter/1
  sensing voltage1/1(V) -> Scope/1  "Inv1"
  connections:
  Solar Cell/RConn1 -- Average-Value DC-DC Converter/LConn3 -- sensing voltage/RConn1 -- ERef/LConn1
  sensing voltage/LConn1 -- Average-Value DC-DC Converter/LConn2 -- Sensing Current/RConn1
  Solar Cell/LConn2 -- Sensing Current/LConn1
  Average-Value DC-DC Converter/LConn1 -- Simulink-PS Converter1/RConn1
  Solar Cell/LConn1 -- Simulink-PS Converter/RConn1
  Average-Value DC-DC Converter/RConn2 -- sensing voltage1/RConn1 -- -/RConn1 -- Capacitor/RConn1
  Average-Value DC-DC Converter/RConn1 -- sensing voltage1/LConn1 -- +/RConn1 -- Capacitor/LConn1

== system scd3busMicrogridDroopControlFidelityLevels/Droop Controller Inverter1/DQ Voltage Reference ==
  freq_cmd : Inport
  V_cmd : Inport  Port=2
  Gain : Gain  Gain=2*pi
  Integrator : Integrator
  Product : Product
  Product1 : Product
  Trigonometric Function : Trigonometry
  Trigonometric Function1 : Trigonometry  Operator=cos
  Vd_ref : Outport
  Vq_ref : Outport  Port=2
  wires:
  Gain/1 -> Integrator/1
  Trigonometric Function1/1 -> Product1/2
  freq_cmd/1 -> Gain/1
  Integrator/1 -> Trigonometric Function1/1, Trigonometric Function/1
  V_cmd/1 -> Product1/1, Product/2
  Trigonometric Function/1 -> Product/1
  Product1/1 -> Vd_ref/1  "Vd_ref"
  Product/1 -> Vq_ref/1  "Vq_ref"

== system scd3busMicrogridDroopControlFidelityLevels/Inverter 1/Averaged Inverter ==
  Averaged Inverter : ee_lib/Semiconductors & Converters/Converters/Converter (Three-Phase)  port_option=ee.enum.threePhasePort.expanded  fidelity_option=ee.enum.converters.fidelity.detailed  device_type=ee.enum.converters.switchingdevice.averaged  showThermalPort=false  K=0  Vth=0.5 V  Vgt=1e-3 V  Vgt_off=-1 V  Ih=1 A  Vf=0.8 V  Ron=1.0000e-03 Ohm  Rds=0.001 Ohm  Goff=2.0000e-04 1/Ohm  Eon_scalar=22.86e-3 J  Eoff_scalar=17.14e-3 J  Eoff_natural_commutation=10e-3 J  Voff=300 V  Iout_scalar=600 A  onCurrentMeasDelay=0 s  useCurrentFromPreviousCycle=false  useVoltageFromPreviousCycle=false  diode_param=ee.enum.converters.protectiondiode.nodynamics  diode_Vf=0.8 V  diode_Ron=0.001 Ohm  diode_Goff=1e-5 1/Ohm  diode_C=50 nF  diode_iRM=-235 A  diode_iF=300 A  diode_idot=-50 A/us  diode_trr_param=ee.enum.converters.diodetrr.trr_factor  diode_trr_factor=3  diode_trr=15 us  diode_Qrr=1.5e+3 s*uA  diode_rec_loss_model=ee.enum.diode.reverseRecoveryModel.fixed  diode_ErecVal=0 J  diode_scaleWithIandV=false  diode_ErecMat=zeros(2, 3) J  diode_TjrecVec=[298.15, 398.15] K  diode_IfrecVec=[.1, 1, 10] A  diode_IrecVal=10 A  diode_VrecVal=10 V  diode_tFilter=1 / 1000 / 100 s  thermal_network_parameterization=ee.enum.thermalNetworkTopology.external  Rth=[.08, .5] K/W  Rth_Cauer=[.08, .1, .5] K/W  Rth_Foster=[.08, .14, .22, .16] K/W  thermal_mass_parameterization=ee.enum.thermalNetwork.timeconstant  thermal_mass=[.01, .5] J/K  thermal_mass_Cauer=[.01, .1, .5] J/K  thermal_mass_Foster=[.001, .005, .05, .5] J/K  thermal_time_constant=[.001, .2] s  thermal_time_constant_Cauer=[.001, .1, .2] s  thermal_time_constant_Foster=[7e-05, .0007, .01, .08] s  thermal_mass_initial_temperatures=[25, 25] degC  thermal_mass_initial_temperatures_Cauer=[25, 25, 25] degC  junction_thermal_mass=0.01 J/K  Tvec_initial_Foster=[25, 25, 25, 25] degC  snubber_type=ee.enum.converters.snubber.exclude  Cs=1e-7 F  Rs=0.1 Ohm  Vce_loss=[0, 150, 300] V
      settings: InternalSimscapePortConfiguration="{\"Bottom\":[],\"Left\":[{\"id\":\"G\",\"label\":\"G\",\"type\":\"foundation.electrical.twelve_phase\"},{\"id\":\"a\",\"label\":\"a\",\"type\":\"foundation.electrical.electrical\"},{\"id\":\"b\",\"label\":\"b\",\"type\":\"foundation.electrical.electrical\"},{\"id\":\"c\",\"label\":\"c\",\"type\":\"foundation.electrical.electrical\"}],\"Right\":[{\"id\":\"p\",\"label\":\"+\",\"type\":\"foundation.electrical.electrical\"},{\"id\":\"n\",\"label\":\"-\",\"type\":\"foundation.electrical.electrical\"}],\"Top\":[]}"
  + : PMIOPort  Side=Right
  G : PMIOPort  Port=2  Side=Left
  a : PMIOPort  Port=3  Side=Left
  b : PMIOPort  Port=4  Side=Left
  - : PMIOPort  Port=5  Side=Right
  c : PMIOPort  Port=6  Side=Left
  connections:
  c/RConn1 -- Averaged Inverter/LConn4
  a/RConn1 -- Averaged Inverter/LConn2
  G/RConn1 -- Averaged Inverter/LConn1
  -/RConn1 -- Averaged Inverter/RConn2
  b/RConn1 -- Averaged Inverter/LConn3
  +/RConn1 -- Averaged Inverter/RConn1

== system scd3busMicrogridDroopControlFidelityLevels/Inverter 1/IGBT Inverter ==
  IGBT Inverter : ee_lib/Semiconductors & Converters/Converters/Converter (Three-Phase)  port_option=ee.enum.threePhasePort.expanded  fidelity_option=ee.enum.converters.fidelity.detailed  device_type=ee.enum.converters.switchingdevice.igbt  showThermalPort=false  K=0  Vth=0.5 V  Vgt=1e-3 V  Vgt_off=-1 V  Ih=1 A  Vf=0.8 V  Ron=1.0000e-03 Ohm  Rds=0.001 Ohm  Goff=2.0000e-04 1/Ohm  Eon_scalar=22.86e-3 J  Eoff_scalar=17.14e-3 J  Eoff_natural_commutation=10e-3 J  Voff=300 V  Iout_scalar=600 A  onCurrentMeasDelay=0 s  useCurrentFromPreviousCycle=false  useVoltageFromPreviousCycle=false  diode_param=ee.enum.converters.protectiondiode.nodynamics  diode_Vf=0.8 V  diode_Ron=0.001 Ohm  diode_Goff=1e-5 1/Ohm  diode_C=50 nF  diode_iRM=-235 A  diode_iF=300 A  diode_idot=-50 A/us  diode_trr_param=ee.enum.converters.diodetrr.trr_factor  diode_trr_factor=3  diode_trr=15 us  diode_Qrr=1.5e+3 s*uA  diode_rec_loss_model=ee.enum.diode.reverseRecoveryModel.fixed  diode_ErecVal=0 J  diode_scaleWithIandV=false  diode_ErecMat=zeros(2, 3) J  diode_TjrecVec=[298.15, 398.15] K  diode_IfrecVec=[.1, 1, 10] A  diode_IrecVal=10 A  diode_VrecVal=10 V  diode_tFilter=1 / 1000 / 100 s  thermal_network_parameterization=ee.enum.thermalNetworkTopology.external  Rth=[.08, .5] K/W  Rth_Cauer=[.08, .1, .5] K/W  Rth_Foster=[.08, .14, .22, .16] K/W  thermal_mass_parameterization=ee.enum.thermalNetwork.timeconstant  thermal_mass=[.01, .5] J/K  thermal_mass_Cauer=[.01, .1, .5] J/K  thermal_mass_Foster=[.001, .005, .05, .5] J/K  thermal_time_constant=[.001, .2] s  thermal_time_constant_Cauer=[.001, .1, .2] s  thermal_time_constant_Foster=[7e-05, .0007, .01, .08] s  thermal_mass_initial_temperatures=[25, 25] degC  thermal_mass_initial_temperatures_Cauer=[25, 25, 25] degC  junction_thermal_mass=0.01 J/K  Tvec_initial_Foster=[25, 25, 25, 25] degC  snubber_type=ee.enum.converters.snubber.exclude  Cs=1e-7 F  Rs=0.1 Ohm  Vce_loss=[0, 150, 300] V
      settings: InternalSimscapePortConfiguration="{\"Bottom\":[],\"Left\":[{\"id\":\"G\",\"label\":\"G\",\"type\":\"foundation.electrical.twelve_phase\"},{\"id\":\"a\",\"label\":\"a\",\"type\":\"foundation.electrical.electrical\"},{\"id\":\"b\",\"label\":\"b\",\"type\":\"foundation.electrical.electrical\"},{\"id\":\"c\",\"label\":\"c\",\"type\":\"foundation.electrical.electrical\"}],\"Right\":[{\"id\":\"p\",\"label\":\"+\",\"type\":\"foundation.electrical.electrical\"},{\"id\":\"n\",\"label\":\"-\",\"type\":\"foundation.electrical.electrical\"}],\"Top\":[]}"
  + : PMIOPort  Side=Right
  G : PMIOPort  Port=2  Side=Left
  a : PMIOPort  Port=3  Side=Left
  b : PMIOPort  Port=4  Side=Left
  - : PMIOPort  Port=5  Side=Right
  c : PMIOPort  Port=6  Side=Left
  connections:
  +/RConn1 -- IGBT Inverter/RConn1
  b/RConn1 -- IGBT Inverter/LConn3
  -/RConn1 -- IGBT Inverter/RConn2
  G/RConn1 -- IGBT Inverter/LConn1
  a/RConn1 -- IGBT Inverter/LConn2
  c/RConn1 -- IGBT Inverter/LConn4

== system scd3busMicrogridDroopControlFidelityLevels/Inverter 2/Average-Value Signal1 ==
  ModWave : Inport
  Bias : Bias  Bias=1  SaturateOnIntegerOverflow=off
  Bias1 : Bias  Bias=1  SaturateOnIntegerOverflow=off
  Gain : Gain  Gain=-1
  Mod. Index1 : Gain  Gain=0.5
  Mux : Mux  Inputs=2
  Rate Transition : RateTransition  OutPortSampleTime=Ts_V
  Selector4 : Selector  InputPortWidth=6  IndexOptions=Index vector (dialog)  Indices=[1 4 2 5 3 6]  OutputSizes=1
  DutyCycle : Outport
  wires:
  ModWave/1 -> Rate Transition/1
  Gain/1 -> Bias1/1
  Mod. Index1/1 -> Gain/1, Mux/1
  Bias/1 -> Mod. Index1/1
  Rate Transition/1 -> Bias/1
  Selector4/1 -> DutyCycle/1
  Bias1/1 -> Mux/2
  Mux/1 -> Selector4/1
